simulink model "Motor_Pos"  (R2026a)
settings: Solver=VariableStepAuto  StopTime=30  FixedStep=0.01
values from neighbouring files (symbols this model uses):
  J = sqrt( (1/length(yReal))*sum(ySim(1:length(yReal))-yReal  ).^2  )    [FOPDT_sysID.m]
undefined symbols (not defined in the file or in its folder): b, gamma, K, L, R, VCC
settings Model: Creator=sansh  LastModifiedBy=jairoviola

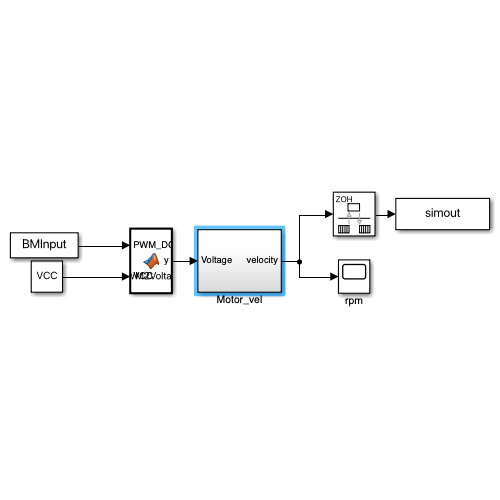
[thumbnail: Simulink's stored preview of the top-level diagram]
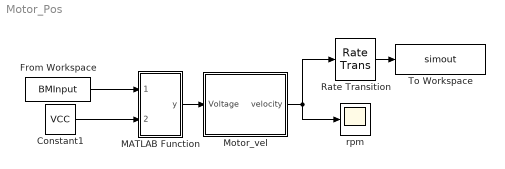
== system Motor_Pos ==
  Constant1 : Constant  Value=VCC
  From Workspace : FromWorkspace  VariableName=BMInput
  MATLAB Function : MATLAB Function  TreatAsAtomicUnit=on
  Motor_vel : Subsystem
  Rate Transition : RateTransition  OutPortSampleTime=0.1
  To Workspace : ToWorkspace  VariableName=simout  SampleTime=-1
  rpm : Scope
      settings: ActiveDisplayYMinimum=-351.24304709260639  ActiveDisplayYMaximum=351.24304709260633
  wires:
  Motor_vel/1(velocity) -> rpm/1, Rate Transition/1
  Constant1/1 -> MATLAB Function/2(VCC)
  From Workspace/1 -> MATLAB Function/1(PWM_DC)
  MATLAB Function/1(y) -> Motor_vel/1(Voltage)
  Rate Transition/1 -> To Workspace/1

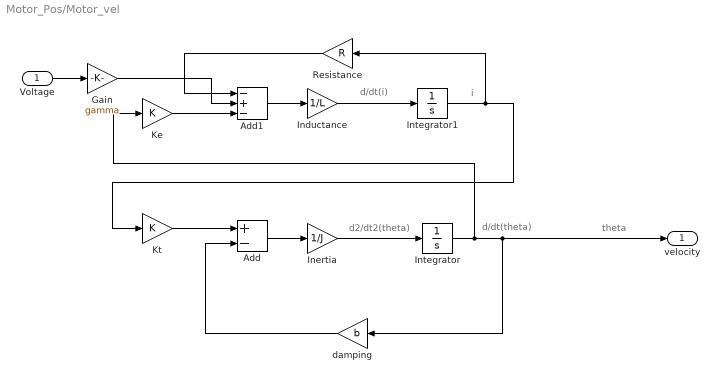
== system Motor_Pos/Motor_vel ==
  note: i
  note: d/dt(i)
  note: d2/dt2(theta)
  note: d/dt(theta)
  note: theta
  Voltage : Inport
  Add : Sum  Inputs=+-
  Add1 : Sum  Inputs=-+-
  Gain : Gain  Gain=gamma
  Inductance : Gain  Gain=1/L
  Inertia : Gain  Gain=1/J
  Integrator : Integrator
  Integrator1 : Integrator
  Ke : Gain  Gain=K
  Kt : Gain  Gain=K
  Resistance : Gain  Gain=R
  damping : Gain  Gain=b
  velocity : Outport
  wires:
  Inertia/1 -> Integrator/1
  Inductance/1 -> Integrator1/1
  Integrator1/1 -> Resistance/1, Kt/1
  Voltage/1 -> Gain/1
  Add/1 -> Inertia/1
  damping/1 -> Add/2
  Kt/1 -> Add/1
  Resistance/1 -> Add1/1
  Ke/1 -> Add1/3
  Add1/1 -> Inductance/1
  Integrator/1 -> Ke/1, velocity/1, damping/1
  Gain/1 -> Add1/2

== matlab function Motor_Pos/MATLAB Function ==
  data: PWM_DC input; y output; VCC input
function y = PWM2Voltage(PWM_DC,VCC)

y=PWM_DC*VCC/255;



end
